simulink model "StepByStep_Article"  (R2014b)
settings: Solver=ode45  StartTime=0.0  StopTime=150  RelTol=1e-3
undefined symbols (not defined in the file or in its folder): A, B, C, D
settings Model: Creator=uidd7441  LastModifiedBy=uidd7441

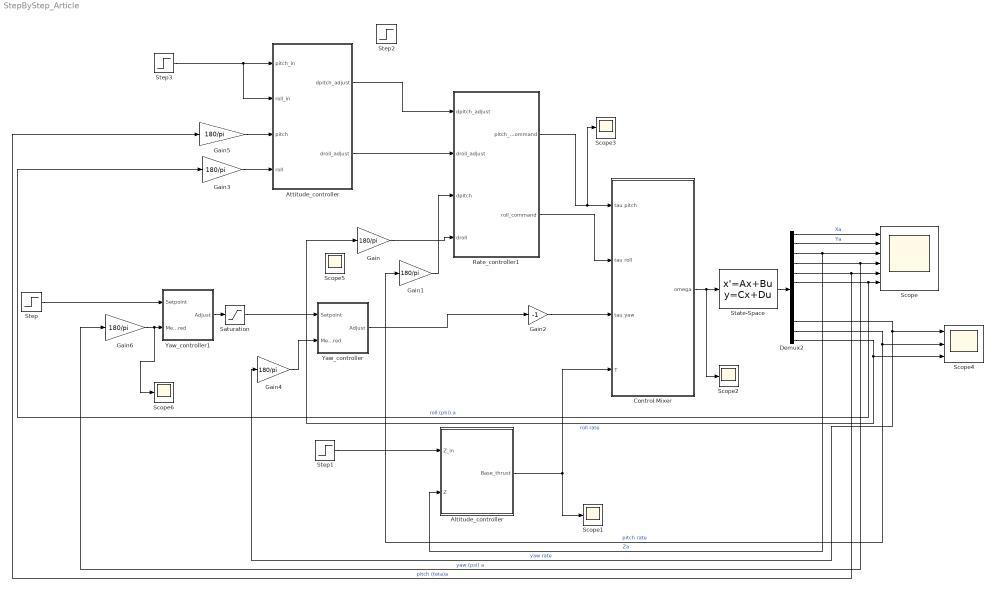
== system StepByStep_Article ==
  Altitude_controller : Subsystem
  Attitude_controller : Subsystem
  Control Mixer : Subsystem  AncestorBlock=roblocks/Dynamics/Control Mixer 4
      mask help: Quadrotor control mixer
      mask Help:
      | Determine rotor speeds based on desired torques and thrust.
      | 
      | <b>Inputs::</b>
      | 
      | tau pitch (1x1)  desired pitching torque [Nm]
      | tau roll (1x1)   desired rolling torque [Nm]
      | tau yaw (1x1)    desired yawing torque [Nm]
      | T (1x1)          desired thrust [N]
      | 
      | <b>Outputs::</b>
      | 
      | w1 (1x1) angular velocity of rotor 1 [rad]
      | w2 (1x1) angular velocity of rotor 2 [rad]
      | w3 (1x1) angular velocity of rotor 3 [rad]
      | w4 (1x1) angular velocity of rotor 4 [rad]
      | 
      | <b>Notes::</b>
      | 
      | - Assumes the rotor labelling convention of RVC Fig 4.16.
      | - The quadrotor is underactuated and has only 4 inputs.
  Demux2 : Demux  Outputs=12
  Gain{,1,3..6} (6 alike) : Gain  Gain=180/pi
  Gain2 : Gain  Gain=-1
  Rate_controller1 : Subsystem
  Saturation : Saturate  UpperLimit=200  LowerLimit=-200
  Scope : Scope  NumInputPorts=6
      settings: YMin=-5~-5~-5~-5~-5~-5  YMax=5~5~5~5~5~5
  Scope{1..3,5..6} (5 alike) : Scope
      Scope1 settings: SaveName=ScopeData2
      Scope2 settings: SaveName=ScopeData3
      Scope3 settings: SaveName=ScopeData4
      Scope5 settings: SaveName=ScopeData6
      Scope6 settings: SaveName=ScopeData11
  Scope4 : Scope  NumInputPorts=3
      settings: YMin=-5~-5~-5  YMax=5~5~5  SaveName=ScopeData5
  State-Space : StateSpace  A=A  B=B  C=C  D=D  X0=[0 0 0 0 0 0 0 0 0 0 0 0]'
  Step : Step  Time=0  After=0  SampleTime=0
  Step1 : Step  Time=0  SampleTime=0
  Step2 : Step  Time=0  SampleTime=0
  Step3 : Step  Time=0  SampleTime=0
  Yaw_controller : Subsystem
  Yaw_controller1 : Subsystem
  wires:
  State-Space/1 -> Demux2/1
  Control Mixer/1(omega) -> Scope2/1, State-Space/1
  Step1/1 -> Altitude_controller/1(Z_in)
  Altitude_controller/1(Base_thrust) -> Control Mixer/4(T), Scope1/1
  Rate_controller1/1(pitch_command) -> Scope3/1, Control Mixer/1(tau pitch)
  Rate_controller1/2(roll_command) -> Control Mixer/2(tau roll)
  Gain2/1 -> Control Mixer/3(tau yaw)
  Demux2/12 -> Scope4/3, Gain/1  "roll rate"
  Demux2/11 -> Scope4/2, Gain1/1  "pitch rate"
  Demux2/2 -> Scope/2  "Ya"
  Demux2/1 -> Scope/1  "Xa"
  Demux2/3 -> Altitude_controller/2(Z), Scope/3  "Za"
  Demux2/4 -> Gain6/1, Scope/4  "yaw (psi) a"
  Demux2/5 -> Gain5/1, Scope/5  "pitch (teta)a"
  Gain/1 -> Rate_controller1/4(droll)
  Gain1/1 -> Rate_controller1/3(dpitch)
  Yaw_controller/1(Adjust) -> Gain2/1
  Gain4/1 -> Yaw_controller/2(Measured)
  Demux2/10 -> Scope4/1, Gain4/1  "yaw rate"
  Gain6/1 -> Scope6/1, Yaw_controller1/2(Measured)
  Demux2/6 -> Gain3/1, Scope/6  "roll (phi) a"
  Step/1 -> Yaw_controller1/1(Setpoint)
  Yaw_controller1/1(Adjust) -> Saturation/1
  Saturation/1 -> Yaw_controller/1(Setpoint)
  Gain5/1 -> Attitude_controller/3(pitch)
  Gain3/1 -> Attitude_controller/4(roll)
  Step3/1 -> Attitude_controller/2(roll_in), Attitude_controller/1(pitch_in)
  Attitude_controller/1(dpitch_adjust) -> Rate_controller1/1(dpitch_adjust)
  Attitude_controller/2(droll_adjust) -> Rate_controller1/2(droll_adjust)

== system StepByStep_Article/Altitude_controller ==
  Z_in : Inport
  Z : Inport  Port=2
  "Min_thrust " : Constant  Value=0  SampleTime=0
  PID_Altitude : Subsystem
  Saturation : Saturate  UpperLimit=60000  LowerLimit=-20000
  Saturation1 : Saturate  UpperLimit=15000  LowerLimit=-20000
  Sum3 : Sum  Inputs=|++
  Base_thrust : Outport
  wires:
  PID_Altitude/1(Adjust) -> Saturation1/1
  Saturation1/1 -> Sum3/1
  Z_in/1 -> PID_Altitude/1(Setpoint)
  Z/1 -> PID_Altitude/2(Measured)
  Sum3/1 -> Saturation/1
  "Min_thrust "/1 -> Sum3/2
  Saturation/1 -> Base_thrust/1

== system StepByStep_Article/Attitude_controller ==
  pitch_in : Inport
  roll_in : Inport  Port=2
  pitch : Inport  Port=3
  roll : Inport  Port=4
  PID_Pitch1 : Subsystem
  PID_Pitch3 : Subsystem
  PID_Roll_Rate1 : Subsystem
  PID_Roll_Rate2 : Subsystem
  dpitch_adjust : Outport
  droll_adjust : Outport  Port=2
  wires:
  PID_Roll_Rate2/1(Adjust) -> dpitch_adjust/1
  pitch/1 -> PID_Roll_Rate2/2(Measured)
  pitch_in/1 -> PID_Roll_Rate2/1(Setpoint)
  PID_Roll_Rate1/1(Adjust) -> droll_adjust/1
  roll/1 -> PID_Roll_Rate1/2(Measured)
  roll_in/1 -> PID_Roll_Rate1/1(Setpoint)

== system StepByStep_Article/Control Mixer ==
  tau pitch : Inport
  tau roll : Inport  Port=2
  tau yaw : Inport  Port=3
  T : Inport  Port=4
  Configuration_X1 : Subsystem
  Configuration_X2 : Subsystem
  Mux1 : Mux
  omega : Outport
  wires:
  Mux1/1 -> omega/1
  T/1 -> Configuration_X1/4(Tau)
  tau yaw/1 -> Configuration_X1/3(Yaw)
  tau roll/1 -> Configuration_X1/2(Roll)
  tau pitch/1 -> Configuration_X1/1(Pitch)
  Configuration_X1/4(W4) -> Mux1/4
  Configuration_X1/3(W3) -> Mux1/3
  Configuration_X1/2(W2) -> Mux1/2
  Configuration_X1/1(W1) -> Mux1/1

== system StepByStep_Article/Rate_controller1 ==
  dpitch_adjust : Inport
  droll_adjust : Inport  Port=2
  dpitch : Inport  Port=3
  droll : Inport  Port=4
  PID_Pitch_Rate1 : Subsystem
  PID_Pitch_Rate3 : Subsystem
  PID_Roll_Rate1 : Subsystem
  PID_Roll_Rate3 : Subsystem
  pitch_command : Outport
  roll_command : Outport  Port=2
  wires:
  dpitch_adjust/1 -> PID_Roll_Rate3/1(Setpoint)
  PID_Roll_Rate3/1(Adjust) -> pitch_command/1
  droll_adjust/1 -> PID_Roll_Rate1/1(Setpoint)
  droll/1 -> PID_Roll_Rate1/2(Measured)
  PID_Roll_Rate1/1(Adjust) -> roll_command/1
  dpitch/1 -> PID_Roll_Rate3/2(Measured)

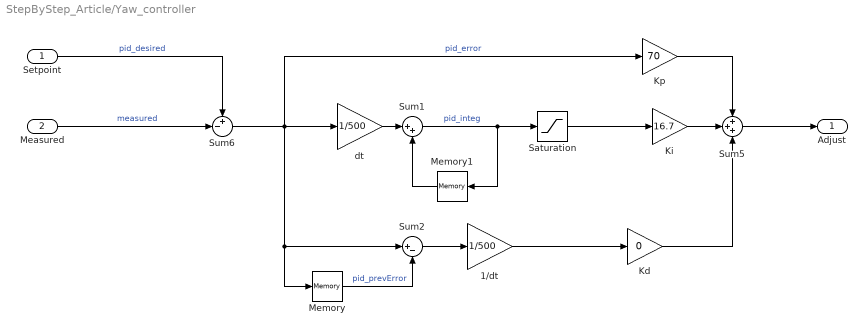
== system StepByStep_Article/Yaw_controller ==
  Setpoint : Inport
  Measured : Inport  Port=2
  1/dt : Gain  Gain=1/500  OutMin=[-200]  OutMax=[200]
  Kd : Gain  Gain=0  OutMin=[-200]  OutMax=[200]
  Ki : Gain  Gain=16.7  OutMin=[-200]  OutMax=[200]
  Kp : Gain  Gain=70  OutMin=[-200]  OutMax=[200]
  Memory : Memory
  Memory1 : Memory
  Saturation : Saturate  UpperLimit=166.7  LowerLimit=-166.7
  Sum1 : Sum  Inputs=|++
  Sum2 : Sum  Inputs=|+-
  Sum5 : Sum  Inputs=+++
  Sum6 : Sum  Inputs=+-|
  dt : Gain  Gain=1/500  OutMin=[-200]  OutMax=[200]
  Adjust : Outport
  wires:
  Saturation/1 -> Ki/1
  Memory1/1 -> Sum1/2
  Sum1/1 -> Saturation/1, Memory1/1  "pid_integ"
  Sum6/1 -> Kp/1, dt/1, Memory/1, Sum2/1  "pid_error"
  1/dt/1 -> Kd/1
  Sum2/1 -> 1/dt/1
  dt/1 -> Sum1/1
  Kd/1 -> Sum5/3
  Kp/1 -> Sum5/1
  Sum5/1 -> Adjust/1
  Ki/1 -> Sum5/2
  Memory/1 -> Sum2/2  "pid_prevError"
  Setpoint/1 -> Sum6/1  "pid_desired"
  Measured/1 -> Sum6/2  "measured"

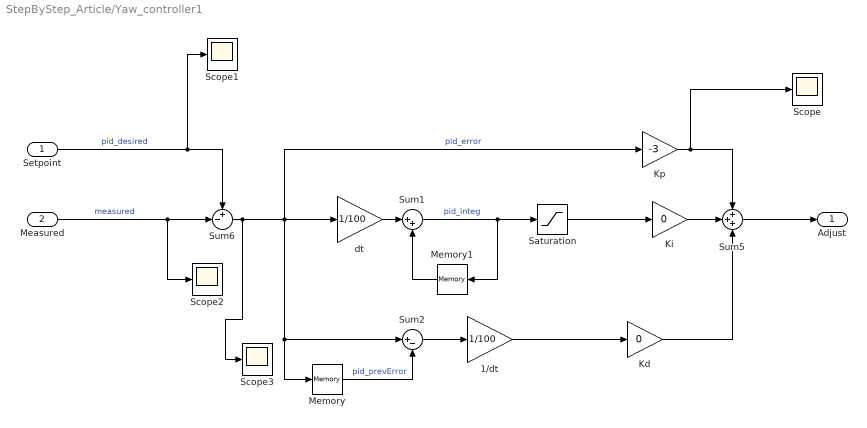
== system StepByStep_Article/Yaw_controller1 ==
  Setpoint : Inport
  Measured : Inport  Port=2
  1/dt : Gain  Gain=1/100  OutMin=[-200]  OutMax=[200]
  Kd : Gain  Gain=0  OutMin=[-200]  OutMax=[200]
  Ki : Gain  Gain=0  OutMin=[-200]  OutMax=[200]
  Kp : Gain  Gain=-3  OutMin=[-200]  OutMax=[200]
  Memory : Memory
  Memory1 : Memory
  Saturation : Saturate  UpperLimit=166.7  LowerLimit=-166.7
  Scope{,1..3} (4 alike) : Scope
      Scope settings: SaveName=ScopeData7
      Scope1 settings: SaveName=ScopeData8
      Scope2 settings: SaveName=ScopeData9
      Scope3 settings: SaveName=ScopeData10
  Sum1 : Sum  Inputs=|++
  Sum2 : Sum  Inputs=|+-
  Sum5 : Sum  Inputs=+++
  Sum6 : Sum  Inputs=+-|
  dt : Gain  Gain=1/100  OutMin=[-200]  OutMax=[200]
  Adjust : Outport
  wires:
  Saturation/1 -> Ki/1
  Memory1/1 -> Sum1/2
  Sum1/1 -> Saturation/1, Memory1/1  "pid_integ"
  Sum6/1 -> Scope3/1, Kp/1, dt/1, Memory/1, Sum2/1  "pid_error"
  1/dt/1 -> Kd/1
  Sum2/1 -> 1/dt/1
  dt/1 -> Sum1/1
  Kd/1 -> Sum5/3
  Kp/1 -> Scope/1, Sum5/1
  Sum5/1 -> Adjust/1
  Ki/1 -> Sum5/2
  Memory/1 -> Sum2/2  "pid_prevError"
  Setpoint/1 -> Scope1/1, Sum6/1  "pid_desired"
  Measured/1 -> Scope2/1, Sum6/2  "measured"

== system StepByStep_Article/Altitude_controller/PID_Altitude ==
  Setpoint : Inport
  Measured : Inport  Port=2
  Derivative : Derivative
  Integrator Limited : Integrator  LimitOutput=on  UpperSaturationLimit=1000  LowerSaturationLimit=-1000
  Kd : Gain  Gain=9000  OutMin=[-200]  OutMax=[200]
  Ki : Gain  Gain=3500  OutMin=[-200]  OutMax=[200]
  Kp : Gain  Gain=11000  OutMin=[-200]  OutMax=[200]
  Sum5 : Sum  Inputs=+++
  Sum6 : Sum  Inputs=+-|
  Adjust : Outport
  wires:
  Sum5/1 -> Adjust/1
  Measured/1 -> Sum6/2  "measured"
  Setpoint/1 -> Sum6/1  "pid_desired"
  Ki/1 -> Sum5/2
  Kp/1 -> Sum5/1
  Kd/1 -> Sum5/3
  Sum6/1 -> Derivative/1, Integrator Limited/1, Kp/1  "pid_error"
  Integrator Limited/1 -> Ki/1
  Derivative/1 -> Kd/1

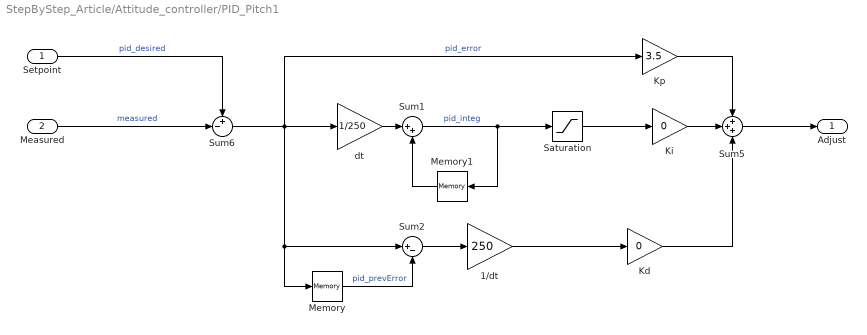
== system StepByStep_Article/Attitude_controller/PID_Pitch1 ==
  Setpoint : Inport
  Measured : Inport  Port=2
  1/dt : Gain  Gain=250  OutMin=[-200]  OutMax=[200]
  Kd : Gain  Gain=0  OutMin=[-200]  OutMax=[200]
  Ki : Gain  Gain=0  OutMin=[-200]  OutMax=[200]
  Kp : Gain  Gain=3.5  OutMin=[-200]  OutMax=[200]
  Memory : Memory
  Memory1 : Memory
  Saturation : Saturate  UpperLimit=20  LowerLimit=-20
  Sum1 : Sum  Inputs=|++
  Sum2 : Sum  Inputs=|+-
  Sum5 : Sum  Inputs=+++
  Sum6 : Sum  Inputs=+-|
  dt : Gain  Gain=1/250  OutMin=[-200]  OutMax=[200]
  Adjust : Outport
  wires:
  Measured/1 -> Sum6/2  "measured"
  Setpoint/1 -> Sum6/1  "pid_desired"
  Memory/1 -> Sum2/2  "pid_prevError"
  Ki/1 -> Sum5/2
  Sum5/1 -> Adjust/1
  Kp/1 -> Sum5/1
  Kd/1 -> Sum5/3
  dt/1 -> Sum1/1
  Sum2/1 -> 1/dt/1
  1/dt/1 -> Kd/1
  Sum6/1 -> Sum2/1, Memory/1, dt/1, Kp/1  "pid_error"
  Sum1/1 -> Memory1/1, Saturation/1  "pid_integ"
  Memory1/1 -> Sum1/2
  Saturation/1 -> Ki/1

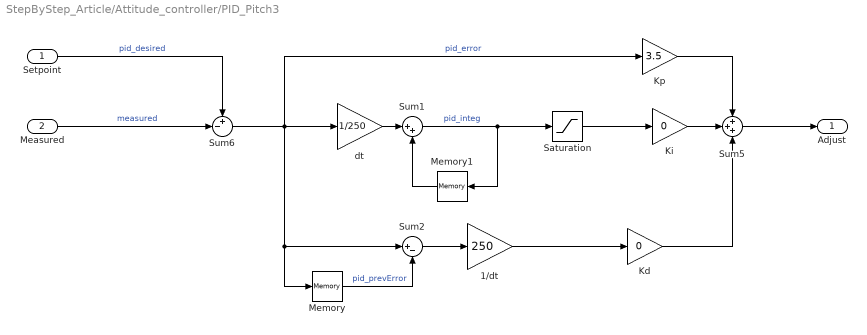
== system StepByStep_Article/Attitude_controller/PID_Pitch3 ==
  Setpoint : Inport
  Measured : Inport  Port=2
  1/dt : Gain  Gain=250  OutMin=[-200]  OutMax=[200]
  Kd : Gain  Gain=0  OutMin=[-200]  OutMax=[200]
  Ki : Gain  Gain=0  OutMin=[-200]  OutMax=[200]
  Kp : Gain  Gain=3.5  OutMin=[-200]  OutMax=[200]
  Memory : Memory
  Memory1 : Memory
  Saturation : Saturate  UpperLimit=20  LowerLimit=-20
  Sum1 : Sum  Inputs=|++
  Sum2 : Sum  Inputs=|+-
  Sum5 : Sum  Inputs=+++
  Sum6 : Sum  Inputs=+-|
  dt : Gain  Gain=1/250  OutMin=[-200]  OutMax=[200]
  Adjust : Outport
  wires:
  Saturation/1 -> Ki/1
  Memory1/1 -> Sum1/2
  Sum1/1 -> Saturation/1, Memory1/1  "pid_integ"
  Sum6/1 -> Kp/1, dt/1, Memory/1, Sum2/1  "pid_error"
  1/dt/1 -> Kd/1
  Sum2/1 -> 1/dt/1
  dt/1 -> Sum1/1
  Kd/1 -> Sum5/3
  Kp/1 -> Sum5/1
  Sum5/1 -> Adjust/1
  Ki/1 -> Sum5/2
  Memory/1 -> Sum2/2  "pid_prevError"
  Setpoint/1 -> Sum6/1  "pid_desired"
  Measured/1 -> Sum6/2  "measured"

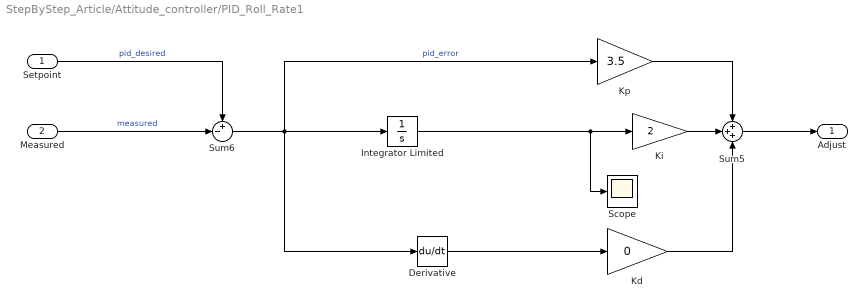
== system StepByStep_Article/Attitude_controller/PID_Roll_Rate1 ==
  Setpoint : Inport
  Measured : Inport  Port=2
  Derivative : Derivative
  Integrator Limited : Integrator  LimitOutput=on  UpperSaturationLimit=20  LowerSaturationLimit=-20
  Kd : Gain  Gain=0  OutMin=[-200]  OutMax=[200]
  Ki : Gain  Gain=2  OutMin=[-200]  OutMax=[200]
  Kp : Gain  Gain=3.5  OutMin=[-200]  OutMax=[200]
  Scope : Scope
  Sum5 : Sum  Inputs=+++
  Sum6 : Sum  Inputs=+-|
  Adjust : Outport
  wires:
  Derivative/1 -> Kd/1
  Integrator Limited/1 -> Ki/1, Scope/1
  Sum6/1 -> Kp/1, Integrator Limited/1, Derivative/1  "pid_error"
  Kd/1 -> Sum5/3
  Kp/1 -> Sum5/1
  Sum5/1 -> Adjust/1
  Ki/1 -> Sum5/2
  Setpoint/1 -> Sum6/1  "pid_desired"
  Measured/1 -> Sum6/2  "measured"

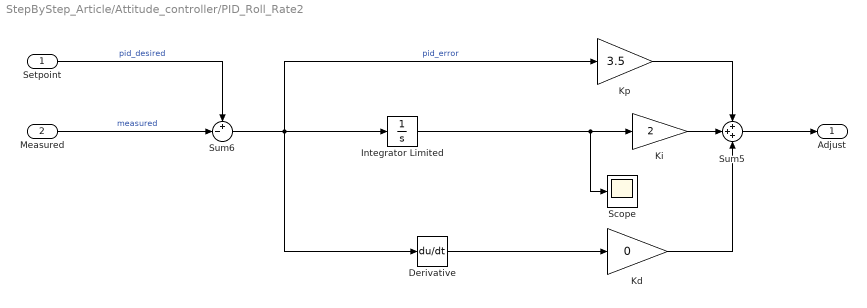
== system StepByStep_Article/Attitude_controller/PID_Roll_Rate2 ==
  Setpoint : Inport
  Measured : Inport  Port=2
  Derivative : Derivative
  Integrator Limited : Integrator  LimitOutput=on  UpperSaturationLimit=20  LowerSaturationLimit=-20
  Kd : Gain  Gain=0  OutMin=[-200]  OutMax=[200]
  Ki : Gain  Gain=2  OutMin=[-200]  OutMax=[200]
  Kp : Gain  Gain=3.5  OutMin=[-200]  OutMax=[200]
  Scope : Scope
  Sum5 : Sum  Inputs=+++
  Sum6 : Sum  Inputs=+-|
  Adjust : Outport
  wires:
  Measured/1 -> Sum6/2  "measured"
  Setpoint/1 -> Sum6/1  "pid_desired"
  Ki/1 -> Sum5/2
  Sum5/1 -> Adjust/1
  Kp/1 -> Sum5/1
  Kd/1 -> Sum5/3
  Sum6/1 -> Derivative/1, Integrator Limited/1, Kp/1  "pid_error"
  Integrator Limited/1 -> Scope/1, Ki/1
  Derivative/1 -> Kd/1

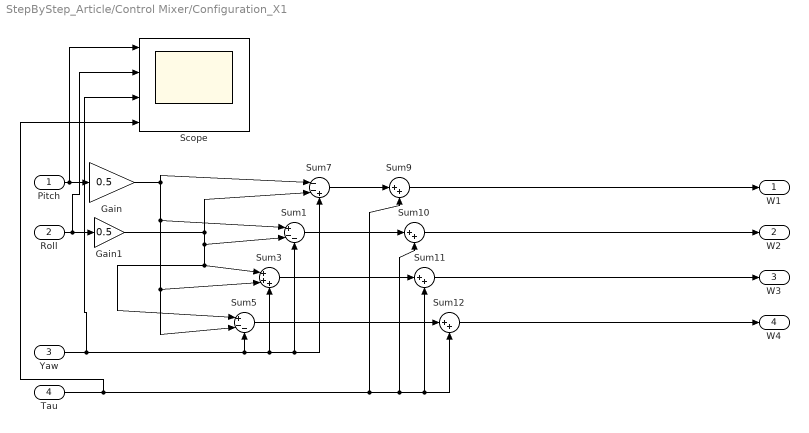
== system StepByStep_Article/Control Mixer/Configuration_X1 ==
  Pitch : Inport
  Roll : Inport  Port=2
  Yaw : Inport  Port=3
  Tau : Inport  Port=4
  Gain : Gain  Gain=0.5
  Gain1 : Gain  Gain=0.5
  Scope : Scope  NumInputPorts=4
      settings: YMin=-5~-5~-5~-5  YMax=5~5~5~5
  Sum1 : Sum  Inputs=|+--  SaturateOnIntegerOverflow=on  InputSameDT=on  OutDataTypeStr=Inherit: Same as first input
  Sum{9..12} (4 alike) : Sum  Inputs=|++  SaturateOnIntegerOverflow=on  InputSameDT=on  OutDataTypeStr=Inherit: Same as first input
  Sum3 : Sum  Inputs=|+++  SaturateOnIntegerOverflow=on  InputSameDT=on  OutDataTypeStr=Inherit: Same as first input
  Sum5 : Sum  Inputs=|+--  SaturateOnIntegerOverflow=on  InputSameDT=on  OutDataTypeStr=Inherit: Same as first input
  Sum7 : Sum  Inputs=|--+  SaturateOnIntegerOverflow=on  InputSameDT=on  OutDataTypeStr=Inherit: Same as first input
  W1 : Outport
  W2 : Outport  Port=2
  W3 : Outport  Port=3
  W4 : Outport  Port=4
  wires:
  Sum12/1 -> W4/1
  Sum11/1 -> W3/1
  Sum10/1 -> W2/1
  Sum9/1 -> W1/1
  Gain1/1 -> Sum3/1, Sum5/1, Sum1/2, Sum7/2
  Gain/1 -> Sum3/2, Sum5/2, Sum1/1, Sum7/1
  Pitch/1 -> Scope/1, Gain/1
  Roll/1 -> Scope/2, Gain1/1
  Sum1/1 -> Sum10/1
  Sum7/1 -> Sum9/1
  Sum5/1 -> Sum12/1
  Tau/1 -> Scope/4, Sum9/2, Sum10/2, Sum12/2, Sum11/2
  Yaw/1 -> Scope/3, Sum1/3, Sum7/3, Sum3/3, Sum5/3
  Sum3/1 -> Sum11/1

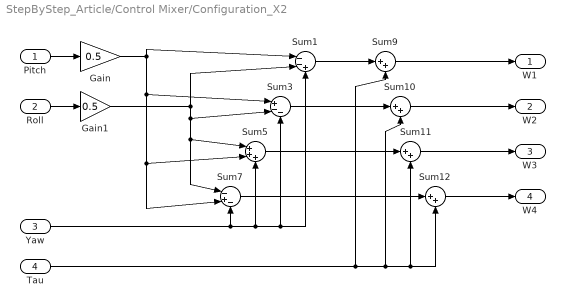
== system StepByStep_Article/Control Mixer/Configuration_X2 ==
  Pitch : Inport
  Roll : Inport  Port=2
  Yaw : Inport  Port=3
  Tau : Inport  Port=4
  Gain : Gain  Gain=0.5
  Gain1 : Gain  Gain=0.5
  Sum1 : Sum  Inputs=|--+  SaturateOnIntegerOverflow=on  InputSameDT=on  OutDataTypeStr=Inherit: Same as first input
  Sum{9..12} (4 alike) : Sum  Inputs=|++  SaturateOnIntegerOverflow=on  InputSameDT=on  OutDataTypeStr=Inherit: Same as first input
  Sum3 : Sum  Inputs=|+--  SaturateOnIntegerOverflow=on  InputSameDT=on  OutDataTypeStr=Inherit: Same as first input
  Sum5 : Sum  Inputs=|+++  SaturateOnIntegerOverflow=on  InputSameDT=on  OutDataTypeStr=Inherit: Same as first input
  Sum7 : Sum  Inputs=|-+-  SaturateOnIntegerOverflow=on  InputSameDT=on  OutDataTypeStr=Inherit: Same as first input
  W1 : Outport
  W2 : Outport  Port=2
  W3 : Outport  Port=3
  W4 : Outport  Port=4
  wires:
  Sum5/1 -> Sum11/1
  Yaw/1 -> Sum7/3, Sum5/3, Sum1/3, Sum3/3
  Tau/1 -> Sum11/2, Sum12/2, Sum10/2, Sum9/2
  Sum7/1 -> Sum12/1
  Sum1/1 -> Sum9/1
  Sum3/1 -> Sum10/1
  Roll/1 -> Gain1/1
  Pitch/1 -> Gain/1
  Gain/1 -> Sum3/1, Sum7/2, Sum5/2, Sum1/1
  Gain1/1 -> Sum1/2, Sum3/2, Sum5/1, Sum7/1
  Sum9/1 -> W1/1
  Sum10/1 -> W2/1
  Sum11/1 -> W3/1
  Sum12/1 -> W4/1

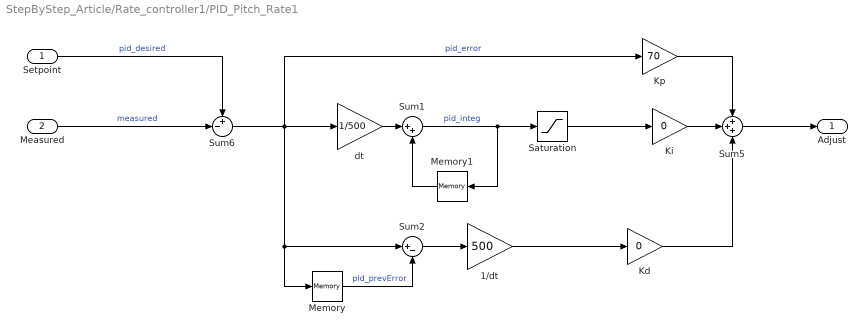
== system StepByStep_Article/Rate_controller1/PID_Pitch_Rate1 ==
  Setpoint : Inport
  Measured : Inport  Port=2
  1/dt : Gain  Gain=500  OutMin=[-200]  OutMax=[200]
  Kd : Gain  Gain=0  OutMin=[-200]  OutMax=[200]
  Ki : Gain  Gain=0  OutMin=[-200]  OutMax=[200]
  Kp : Gain  Gain=70  OutMin=[-200]  OutMax=[200]
  Memory : Memory
  Memory1 : Memory
  Saturation : Saturate  UpperLimit=33  LowerLimit=-33
  Sum1 : Sum  Inputs=|++
  Sum2 : Sum  Inputs=|+-
  Sum5 : Sum  Inputs=+++
  Sum6 : Sum  Inputs=+-|
  dt : Gain  Gain=1/500  OutMin=[-200]  OutMax=[200]
  Adjust : Outport
  wires:
  Saturation/1 -> Ki/1
  Memory1/1 -> Sum1/2
  Sum1/1 -> Memory1/1, Saturation/1  "pid_integ"
  Sum6/1 -> Kp/1, dt/1, Memory/1, Sum2/1  "pid_error"
  1/dt/1 -> Kd/1
  Sum2/1 -> 1/dt/1
  dt/1 -> Sum1/1
  Kd/1 -> Sum5/3
  Kp/1 -> Sum5/1
  Sum5/1 -> Adjust/1
  Ki/1 -> Sum5/2
  Memory/1 -> Sum2/2  "pid_prevError"
  Setpoint/1 -> Sum6/1  "pid_desired"
  Measured/1 -> Sum6/2  "measured"

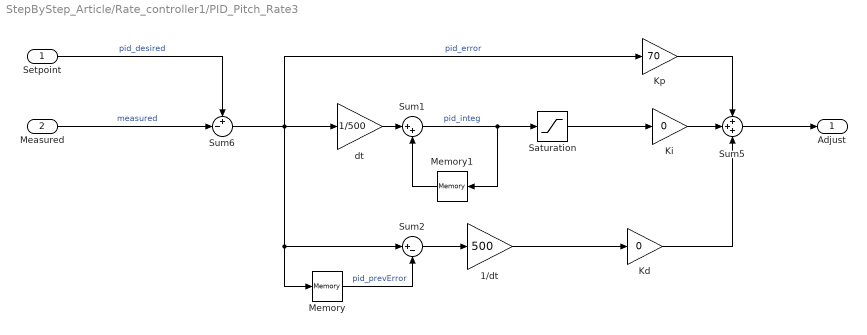
== system StepByStep_Article/Rate_controller1/PID_Pitch_Rate3 ==
  Setpoint : Inport
  Measured : Inport  Port=2
  1/dt : Gain  Gain=500  OutMin=[-200]  OutMax=[200]
  Kd : Gain  Gain=0  OutMin=[-200]  OutMax=[200]
  Ki : Gain  Gain=0  OutMin=[-200]  OutMax=[200]
  Kp : Gain  Gain=70  OutMin=[-200]  OutMax=[200]
  Memory : Memory
  Memory1 : Memory
  Saturation : Saturate  UpperLimit=33  LowerLimit=-33
  Sum1 : Sum  Inputs=|++
  Sum2 : Sum  Inputs=|+-
  Sum5 : Sum  Inputs=+++
  Sum6 : Sum  Inputs=+-|
  dt : Gain  Gain=1/500  OutMin=[-200]  OutMax=[200]
  Adjust : Outport
  wires:
  Measured/1 -> Sum6/2  "measured"
  Setpoint/1 -> Sum6/1  "pid_desired"
  Memory/1 -> Sum2/2  "pid_prevError"
  Ki/1 -> Sum5/2
  Sum5/1 -> Adjust/1
  Kp/1 -> Sum5/1
  Kd/1 -> Sum5/3
  dt/1 -> Sum1/1
  Sum2/1 -> 1/dt/1
  1/dt/1 -> Kd/1
  Sum6/1 -> Sum2/1, Memory/1, dt/1, Kp/1  "pid_error"
  Sum1/1 -> Saturation/1, Memory1/1  "pid_integ"
  Memory1/1 -> Sum1/2
  Saturation/1 -> Ki/1

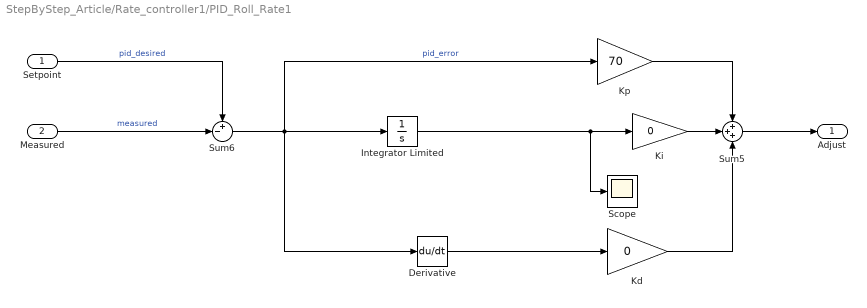
== system StepByStep_Article/Rate_controller1/PID_Roll_Rate1 ==
  Setpoint : Inport
  Measured : Inport  Port=2
  Derivative : Derivative
  Integrator Limited : Integrator  LimitOutput=on  UpperSaturationLimit=1000  LowerSaturationLimit=-1000
  Kd : Gain  Gain=0  OutMin=[-200]  OutMax=[200]
  Ki : Gain  Gain=0  OutMin=[-200]  OutMax=[200]
  Kp : Gain  Gain=70  OutMin=[-200]  OutMax=[200]
  Scope : Scope
  Sum5 : Sum  Inputs=+++
  Sum6 : Sum  Inputs=+-|
  Adjust : Outport
  wires:
  Measured/1 -> Sum6/2  "measured"
  Setpoint/1 -> Sum6/1  "pid_desired"
  Ki/1 -> Sum5/2
  Sum5/1 -> Adjust/1
  Kp/1 -> Sum5/1
  Kd/1 -> Sum5/3
  Sum6/1 -> Derivative/1, Integrator Limited/1, Kp/1  "pid_error"
  Integrator Limited/1 -> Scope/1, Ki/1
  Derivative/1 -> Kd/1

== system StepByStep_Article/Rate_controller1/PID_Roll_Rate3 ==
  Setpoint : Inport
  Measured : Inport  Port=2
  Derivative : Derivative
  Integrator Limited : Integrator  LimitOutput=on  UpperSaturationLimit=1000  LowerSaturationLimit=-1000
  Kd : Gain  Gain=0  OutMin=[-200]  OutMax=[200]
  Ki : Gain  Gain=0  OutMin=[-200]  OutMax=[200]
  Kp : Gain  Gain=70  OutMin=[-200]  OutMax=[200]
  Scope : Scope
  Sum5 : Sum  Inputs=+++
  Sum6 : Sum  Inputs=+-|
  Adjust : Outport
  wires:
  Derivative/1 -> Kd/1
  Integrator Limited/1 -> Ki/1, Scope/1
  Sum6/1 -> Kp/1, Integrator Limited/1, Derivative/1  "pid_error"
  Kd/1 -> Sum5/3
  Kp/1 -> Sum5/1
  Sum5/1 -> Adjust/1
  Ki/1 -> Sum5/2
  Setpoint/1 -> Sum6/1  "pid_desired"
  Measured/1 -> Sum6/2  "measured"
